simulink model "Model_Nagr_Zvezda_treug"  (R2018b)
settings: Solver=VariableStepAuto  StartTime=0.0  StopTime=0.2  RelTol=1e-3
libraries: powerlib x15, peRmsMeasurement x8
settings Model: Creator=sr1  LastModifiedBy=VID Company

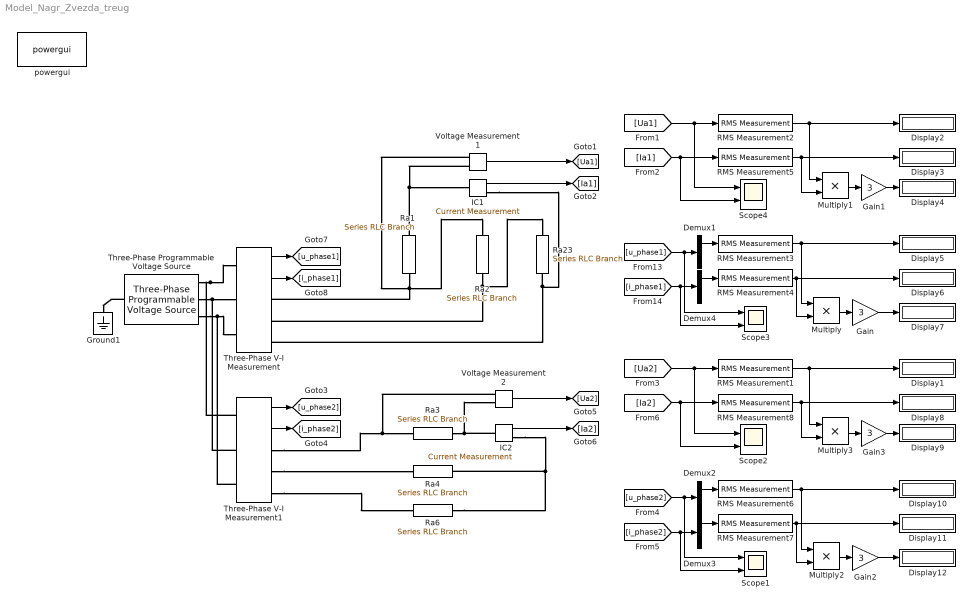
== system Model_Nagr_Zvezda_treug ==
  Demux{1..4} (4 alike) : Demux  Outputs=3
  Display{1..12} (12 alike) : Display
  Gain{,1..3} (4 alike) : Gain  Gain=3
  Ground1 : powerlib/Elements/Ground  LConnTagsString=a
  IC1 : powerlib/Measurements/Current Measurement  PhasorSimulation=off  OutputType=Complex  PSBequivalent=0
  IC2 : powerlib/Measurements/Current Measurement  PhasorSimulation=off  OutputType=Complex  PSBequivalent=0
  Multiply{,1..3} (4 alike) : Product
  RMS Measurement{1..8} (8 alike) : peRmsMeasurement/RMS Measurement  LabelModeActiveChoice=Harmonic  F=50  SpecifyHarmonics=on  K=[1]  Ts=0
  Ra{1..4,6,23} (6 alike) : powerlib/Elements/Series RLC Branch  LConnTagsString=__new0  RConnTagsString=__new0  BranchType=R  Resistance=16  Inductance=1e-3  SetiL0=off  InitialCurrent=0  Capacitance=1e-6  Setx0=off  InitialVoltage=0  Measurements=None
  Scope{1..4} (4 alike) : Scope  NumInputPorts=2
  Three-Phase Programmable Voltage Source : powerlib/Electrical Sources/Three-Phase Programmable Voltage Source  PositiveSequence=[208 0 50]  VariationEntity=None  VariationType=Table of time-amplitude pairs  VariationTypeAlt=Step  VariationStep=0.5  VariationRate=10  VariationMagnitude=0.3  VariationFrequency=2  VariationTiming=[1 2]  VariationPhaseA=off  Amplitudes=[1 0.8 1.2 1.0]  TimeValues=[0 0.1 0.15 0.2]  HarmonicGeneration=off  HarmonicA=[3 0.2 -25 0]  HarmonicB=[2 0.15 35 2]  Timing="[0.05  3]"  BusType=swing  Pref=0  Qref=0  Qmin=-inf  Qmax=inf
  Three-Phase V-I Measurement : powerlib/Measurements/Three-Phase V-I Measurement  VoltageMeasurement=phase-to-ground  SetLabelV=off  LabelV=Vabc  Vpu=off  VpuLL=off  CurrentMeasurement=yes  SetLabelI=off  LabelI=Iabc  Ipu=off  Pbase=100e6  Vbase=500e3  OutputType=Complex  PhasorSimulation=off  PSBequivalent=0
  Three-Phase V-I Measurement1 : powerlib/Measurements/Three-Phase V-I Measurement  VoltageMeasurement=phase-to-ground  SetLabelV=off  LabelV=Vabc  Vpu=off  VpuLL=off  CurrentMeasurement=yes  SetLabelI=off  LabelI=Iabc  Ipu=off  Pbase=100e6  Vbase=500e3  OutputType=Complex  PhasorSimulation=off  PSBequivalent=0
  Voltage Measurement1 : powerlib/Measurements/Voltage Measurement  PhasorSimulation=off  OutputType=Complex  PSBequivalent=0
  Voltage Measurement2 : powerlib/Measurements/Voltage Measurement  PhasorSimulation=off  OutputType=Complex  PSBequivalent=0
  powergui : powerlib/powergui  Priority=1  SimulationMode=Discrete  SampleTime=1e-7  frequency=60  Iterations=50  frequencyindice=50  Pbase=100e6  ErrMax=1e-4  UnitsV=kV  UnitsW=MW  buscounter=0  FunctionMessages=off  echomessages=off  EnableUseOfTLC=off  CurrentSourceSwitches=off  DisableSnubberDevices=off  DisableRonSwitches=off  DisableVfSwitches=off  DisplayEquations=off  SolverType=Tustin/Backward Euler (TBE)  Interpol=off  ExternalGateDelay=off  methode=off  Ts=100  x0status=blocks  SPID=on  SwTol=0  HookPort=off  RestoreLinks=warning  ResistiveCurrentMeasurement=off  Frange=[0:2:500]  Ylog=off  Xlog=on  ShowGrid=off  save=off  variable=ZData  structure=0  ZoomFFT=off  StartTime=0.0  cycles=1  DisplayStyle=1  fundamental=60  FreqAxis=off  MaxFrequency=1000  frequencyindicesteady=1  RmsSteady=1  display=off
  wires:
  Three-Phase V-I Measurement/2 -> [i_phase1]
  Three-Phase V-I Measurement/1 -> [u_phase1]
  RMS Measurement4/1 -> Display6/1, Multiply/2
  [i_phase1] -> Scope3/2, Demux4/1
  [u_phase1] -> Scope3/1, Demux1/1
  Multiply/1 -> Gain/1
  Gain/1 -> Display7/1
  RMS Measurement3/1 -> Display5/1, Multiply/1
  Demux4/1 -> RMS Measurement4/1
  Demux1/1 -> RMS Measurement3/1
  Voltage Measurement1/1 -> [Ua1]
  IC1/1 -> [Ia1]
  [Ia1] -> RMS Measurement5/1, Scope4/2
  Multiply1/1 -> Gain1/1
  Gain1/1 -> Display4/1
  RMS Measurement2/1 -> Display2/1, Multiply1/1
  RMS Measurement5/1 -> Display3/1, Multiply1/2
  [Ua1] -> RMS Measurement2/1, Scope4/1
  Three-Phase V-I Measurement1/1 -> [u_phase2]
  Three-Phase V-I Measurement1/2 -> [i_phase2]
  Voltage Measurement2/1 -> [Ua2]
  IC2/1 -> [Ia2]
  [Ua2] -> RMS Measurement1/1, Scope2/1
  RMS Measurement8/1 -> Display8/1, Multiply3/2
  Multiply2/1 -> Gain2/1
  [Ia2] -> RMS Measurement8/1, Scope2/2
  RMS Measurement6/1 -> Display10/1, Multiply2/1
  RMS Measurement1/1 -> Display1/1, Multiply3/1
  Demux3/1 -> RMS Measurement7/1
  Gain3/1 -> Display9/1
  Demux2/1 -> RMS Measurement6/1
  [u_phase2] -> Scope1/1, Demux2/1
  Multiply3/1 -> Gain3/1
  Gain2/1 -> Display12/1
  RMS Measurement7/1 -> Display11/1, Multiply2/2
  [i_phase2] -> Scope1/2, Demux3/1
  connections:
  Three-Phase Programmable Voltage Source/RConn1 -- Three-Phase V-I Measurement1/LConn1 -- Three-Phase V-I Measurement/LConn1
  Three-Phase Programmable Voltage Source/LConn1 -- Ground1/LConn1
  Three-Phase Programmable Voltage Source/RConn3 -- Three-Phase V-I Measurement1/LConn3 -- Three-Phase V-I Measurement/LConn3
  Three-Phase Programmable Voltage Source/RConn2 -- Three-Phase V-I Measurement1/LConn2 -- Three-Phase V-I Measurement/LConn2
  Ra1/RConn1 -- Three-Phase V-I Measurement/RConn1 -- Voltage Measurement1/LConn1 -- Ra2/LConn1
  Ra2/RConn1 -- Three-Phase V-I Measurement/RConn2 -- Ra23/LConn1
  Ra23/RConn1 -- Three-Phase V-I Measurement/RConn3 -- IC1/RConn1
  Ra1/LConn1 -- Voltage Measurement1/LConn2 -- IC1/LConn1
  Three-Phase V-I Measurement1/RConn2 -- Ra4/LConn1
  Three-Phase V-I Measurement1/RConn1 -- Voltage Measurement2/LConn1 -- Ra3/LConn1
  Three-Phase V-I Measurement1/RConn3 -- Ra6/LConn1
  Ra6/RConn1 -- IC2/RConn1 -- Ra4/RConn1
  Ra3/RConn1 -- Voltage Measurement2/LConn2 -- IC2/LConn1
